simulink model "FOPIDControllerCartPendulum"  (R2022b)
settings: Solver=ode45  StartTime=0.0  StopTime=tfinal  FixedStep=dt  RelTol=1e-3  EnableMultiTasking=on
values from neighbouring files (symbols this model uses):
  A = [4 1 8 6 3 2 5 8 6 7; 4 1 8 6 3 2 5 8 6 7]'    [MainCEoptExample3Ext.m]    (also in MainCEoptExample4.m = sqrt(y0^2 + ((v0+ksi*wn*y0)/w)^2); MainCEoptExample4Ext.m = sqrt(y0^2 + ((v0+ksi*wn*y0)/w)^2); MainCEoptExample8Ext.m = 0.0651; MainCEoptExample8Ext.mat = 0.0651)
  B = m*L    (= 0.05)    [MainCEoptExample8Ext.m]    (also in MainCEoptExample8Ext.mat; TrussConst.m = 1/l*[-c -s c s])
  C = 1/m*[1 2 2 4 4 6 3 7 5 5]'    [MainCEoptExample3Ext.m]    (also in MainCEoptExample6Ext.m = reshape(C  ,size(X)); MainCEoptExample8Ext.m = 2.1; MainCEoptExample8Ext.mat = 2.1)
  dtheta0 = 0.0*pi/180    (= 0)    [MainCEoptExample8Ext.m]    (also in MainCEoptExample8Ext.mat)
  dxdisp0 = 0.0    (= 0)    [MainCEoptExample8Ext.m]    (also in MainCEoptExample8Ext.mat)
  Kd = x(3)    [MainCEoptExample8Ext.m]    (also in MainCEoptExample8Ext.mat = -22.6723976789)
  Ki = x(2)    [MainCEoptExample8Ext.m]    (also in MainCEoptExample8Ext.mat = -5.93575845663)
  Kp = x(1)    [MainCEoptExample8Ext.m]    (also in MainCEoptExample8Ext.mat = -5.17112192449)
  r = 0.0    (= 0)    [MainCEoptExample8Ext.m]    (also in MainCEoptExample8Ext.mat)
  theta0 = x(5)    [MainCEoptExample5.m]    (also in MainCEoptExample5Ext.m; MainCEoptExample8Ext.m = 0.174532925199; MainCEoptExample8Ext.mat = 0.174532925199)
  xdisp0 = 0.0    (= 0)    [MainCEoptExample8Ext.m]    (also in MainCEoptExample8Ext.mat)
libraries: fod x2
settings Model: Creator=julio  LastModifiedBy=americo
settings SolverCC: AlgebraicLoopSolver=TrustRegion
settings DataIOCC: ReturnWorkspaceOutputs=off
settings OptimizationCC: LifeSpan=inf
settings DebuggingCC: UnconnectedInputMsg=warning  UnconnectedOutputMsg=warning  UnconnectedLineMsg=warning  SFUnexpectedBacktrackingDiag=warning  SFNoUnconditionalDefaultTransitionDiag=warning  SFMachineParentedDataDiag=warning  ArithmeticOperatorsInVariantConditions=warning
settings ModelReferenceCC: EnableRefExpFcnMdlSchedulingChecks=on
settings SFSimCC: SimUseLocalCustomCode=off  CustomCodeUndefinedFunction=UseInterfaceOnly
settings RTWCC: RTWUseLocalCustomCode=off
settings CodeAppCC: StateflowObjectComments=on
settings GRTTargetCC: TargetLangStandard=C89/C90 (ANSI)
settings ConfigComp: CovMetricSettings=dw  CovSaveCumulativeToWorkspaceVar=on  CovSaveSingleToWorkspaceVar=on  CovExternalEMLEnable=off

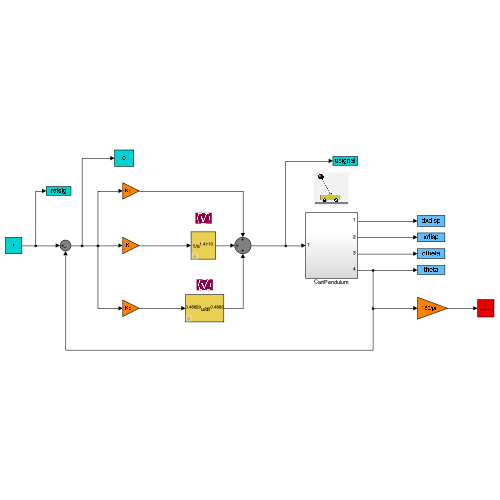
[thumbnail: Simulink's stored preview of the top-level diagram]
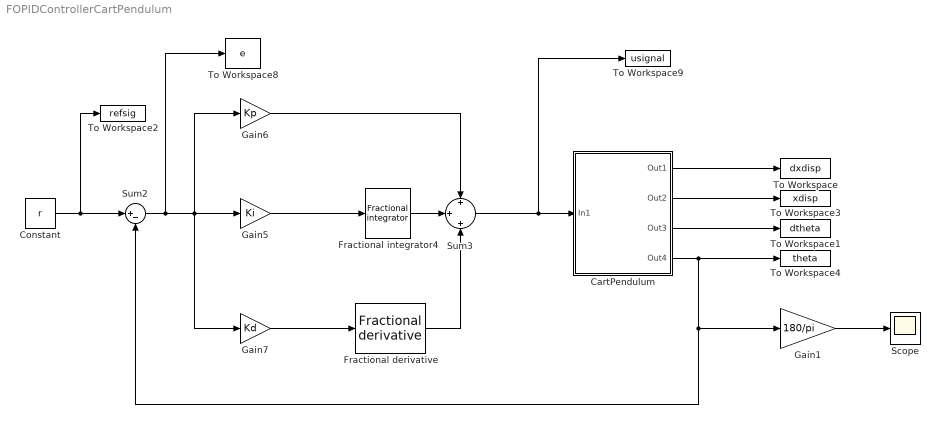
== system FOPIDControllerCartPendulum ==
  CartPendulum : Subsystem
  Constant : Constant  Value=r
  Fractional derivative : fod/Fractional derivative  gam=OrderD  ww=[0.001; 1000]  n=5  nFod=off
      settings: SourceProductName=FOMCON Toolbox
  Fractional integrator4 : fod/Fractional integrator  gam=OrderI  ww=[0.001; 1000]  n=5  nFod=off
      settings: SourceProductName=FOMCON Toolbox
  Gain1 : Gain  Gain=180/pi
  Gain5 : Gain  Gain=Ki
  Gain6 : Gain  Gain=Kp
  Gain7 : Gain  Gain=Kd
  Scope : Scope
  Sum2 : Sum  Inputs=|+-
  Sum3 : Sum  Inputs=+|+|+
  To Workspace : ToWorkspace  VariableName=dxdisp  SampleTime=-1
  To Workspace1 : ToWorkspace  VariableName=dtheta  SampleTime=-1
  To Workspace2 : ToWorkspace  VariableName=refsig  SampleTime=-1
  To Workspace3 : ToWorkspace  VariableName=xdisp  SampleTime=-1
  To Workspace4 : ToWorkspace  VariableName=theta  SampleTime=-1
  To Workspace8 : ToWorkspace  VariableName=e  SampleTime=-1
  To Workspace9 : ToWorkspace  VariableName=usignal  SampleTime=-1
  wires:
  Sum3/1 -> CartPendulum/1(In1), To Workspace9/1
  Gain5/1 -> Fractional integrator4/1
  Gain6/1 -> Sum3/1
  Fractional integrator4/1 -> Sum3/2
  Gain7/1 -> Fractional derivative/1
  Fractional derivative/1 -> Sum3/3
  Sum2/1 -> To Workspace8/1, Gain7/1, Gain6/1, Gain5/1
  CartPendulum/2(Out2) -> To Workspace3/1
  CartPendulum/3(Out3) -> To Workspace1/1
  CartPendulum/4(Out4) -> Gain1/1, Sum2/2, To Workspace4/1
  Gain1/1 -> Scope/1
  CartPendulum/1(Out1) -> To Workspace/1
  Constant/1 -> To Workspace2/1, Sum2/1

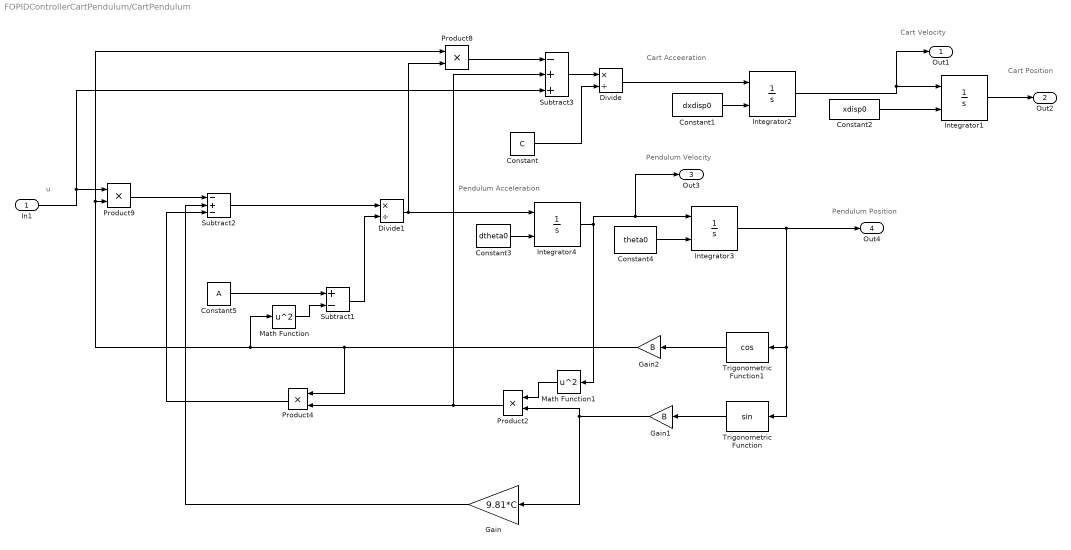
== system FOPIDControllerCartPendulum/CartPendulum ==
  note: u
  note: Pendulum Acceleration
  note: Pendulum Position
  note: Cart Acceeration
  note: Cart Velocity
  note: Cart Position
  note: Pendulum Velocity
  In1 : Inport
  Constant : Constant  Value=C
  Constant1 : Constant  Value=dxdisp0
  Constant2 : Constant  Value=xdisp0
  Constant3 : Constant  Value=dtheta0
  Constant4 : Constant  Value=theta0
  Constant5 : Constant  Value=A
  Divide : Product  Inputs=*/
  Divide1 : Product  Inputs=*/
  Gain : Gain  Gain=9.81*C
  Gain1 : Gain  Gain=B
  Gain2 : Gain  Gain=B
  Integrator{1..4} (4 alike) : Integrator  InitialConditionSource=external
  Math Function : Math  Operator=square  SignedPower=on
  Math Function1 : Math  Operator=square  SignedPower=on
  Product{2,4,8..9} (4 alike) : Product
  Subtract1 : Sum  Inputs=+-
  Subtract2 : Sum  Inputs=-+-
  Subtract3 : Sum  Inputs=-++
  Trigonometric Function : Trigonometry
  Trigonometric Function1 : Trigonometry  Operator=cos
  Out1 : Outport
  Out2 : Outport  Port=2
  Out3 : Outport  Port=3
  Out4 : Outport  Port=4
  wires:
  Integrator4/1 -> Math Function1/1, Out3/1, Integrator3/1
  Gain2/1 -> Product4/1, Math Function/1, Product8/1, Product9/2
  Product9/1 -> Subtract2/1
  Constant2/1 -> Integrator1/2
  Subtract2/1 -> Divide1/1
  Integrator2/1 -> Out1/1, Integrator1/1
  Divide/1 -> Integrator2/1
  Trigonometric Function1/1 -> Gain2/1
  Subtract1/1 -> Divide1/2
  Divide1/1 -> Integrator4/1, Product8/2
  Math Function/1 -> Subtract1/2
  Math Function1/1 -> Product2/1
  Gain1/1 -> Gain/1, Product2/2
  Product8/1 -> Subtract3/1
  Subtract3/1 -> Divide/1
  Product4/1 -> Subtract2/3
  Product2/1 -> Subtract3/2, Product4/2
  In1/1 -> Subtract3/3, Product9/1
  Gain/1 -> Subtract2/2
  Constant/1 -> Divide/2
  Integrator3/1 -> Out4/1, Trigonometric Function/1, Trigonometric Function1/1
  Constant4/1 -> Integrator3/2
  Constant3/1 -> Integrator4/2
  Constant1/1 -> Integrator2/2
  Constant5/1 -> Subtract1/1
  Trigonometric Function/1 -> Gain1/1
  Integrator1/1 -> Out2/1
